simulink model "simulink2"  (R2014a)
settings: Solver=ode45  StartTime=0.0  StopTime=10.0  RelTol=1e-3
values from neighbouring files (symbols this model uses):
  Kc = 800    [Esercizio1.m]    (also in Esercizio2.m = -0.1)
  Kr = 2    [Esercizio1.m]    (also in Esercizio2.m = 0.5)
libraries: simulink x2, cstblocks x1
settings Model: Creator=UTENTE  LastModifiedBy=UTENTE

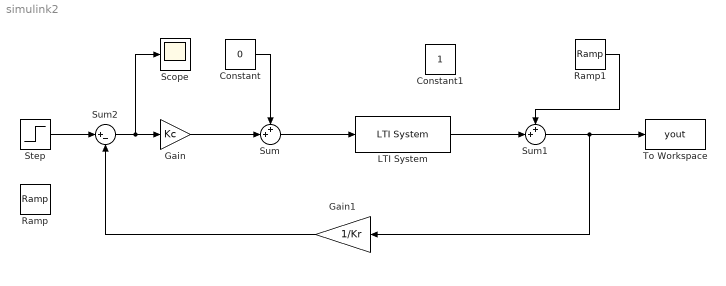
== system simulink2 ==
  Constant : Constant  Value=0
  Constant1 : Constant
  Gain : Gain  Gain=Kc
  Gain1 : Gain  Gain=1/Kr
  LTI System : cstblocks/LTI System  sys=F  IC=[]
  Ramp : simulink/Sources/Ramp  slope=1  start=0  X0=0
  Ramp1 : simulink/Sources/Ramp  slope=0.01  start=0  X0=0
  Scope : Scope
  Step : Step  Time=0  After=2  SampleTime=0
  Sum : Sum  Inputs=++|
  Sum1 : Sum  Inputs=++|
  Sum2 : Sum  Inputs=|+-
  To Workspace : ToWorkspace  VariableName=yout  SaveFormat=Timeseries  SampleTime=-1
  wires:
  Gain/1 -> Sum/2
  Sum/1 -> LTI System/1
  LTI System/1 -> Sum1/2
  Sum1/1 -> Gain1/1, To Workspace/1
  Sum2/1 -> Scope/1, Gain/1
  Step/1 -> Sum2/1
  Gain1/1 -> Sum2/2
  Constant/1 -> Sum/1
  Ramp1/1 -> Sum1/1
